simulink library "visionanalysis"  (R2024b)
settings: Solver=ode45  StartTime=0.0  StopTime=10.0  RelTol=1e-3
undefined symbols (not defined in the file or in its folder): dtInfo, fspecial
libraries: visionstatistics x1
(part 2 of 2)

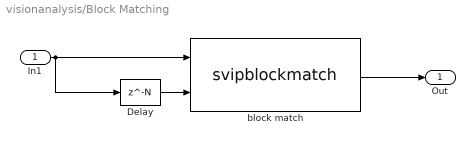
== system visionanalysis/Block Matching ==
  In1 : Inport
  Delay : Delay  DelayLength=N
  block match : S-Function  DialogController=vipDDGCreate  FunctionName=svipblockmatch  Parameters=searchMethod,blockSize,overlapping,maxDisplacement,matchCriteria,outVelForm,dtInfo.prodOutputMode,dtInfo.prodOutputWordLength,dtInfo.prodOutputFracLength,dtInfo.accumMode,dtInfo.accumWordLength,dtInfo.accumFracLength,dtInfo.outputMode,dtInfo.outputWordLength,dtInfo.outputFracLength,dtInfo.roundingMode,dtInfo.overflowMode  SFunctionDeploymentMode=off  EnableBusSupport=off  mask(block match){which2img=Two images, N=1, searchMethod=Exhaustive, blockSize=blockSize, overlapping=overlapping, maxDisplacement=maxDisplacement, matchCriteria=Mean square error (MSE), outVelForm=Magnitude-squared, outputMode=Binary point scaling, outputWordLength=outputWordLength, outputFracLength=outputFracLength, accumMode=Binary point scaling, accumWordLength=accumWordLength, accumFracLength=accumFracLength, prodOutputMode=Binary point scaling, prodOutputWordLength=prodOutputWordLength, prodOutputFracLength=prodOutputFracLength, roundingMode=Floor, overflowMode=on, LockScale=off}
      mask prompts: which2img "Estimate motion between:"; searchMethod "Search method:"; blockSize "Block size [height width]:"; overlapping "Overlap size [r c]:"; maxDisplacement "Maximum displacement [r c]:"; matchCriteria "Block matching criteria:"; outVelForm "Velocity output:"; outputMode "Fixed-point output attributes:"; outputWordLength "Output word length:"; outputFracLength "Output fractional length:"; accumMode "Fixed-point accumulator attributes:"; accumWordLength "Accumulator word length:"; accumFracLength "Accumulator fraction length:"; prodOutputMode "Fixed-point product output attributes:"; prodOutputWordLength "Product output word length:"; prodOutputFracLength "Product output fraction length:"; roundingMode "Round integer calculations towards:"; overflowMode "Saturate on integer overflow"; LockScale "Lock scaling"
      mask help: Estimates motion between two images or two video frames using block matching method.
      mask init:
      | dtInfo = dspGetFixptDataTypeInfo(gcbh,15);
      mask TypeOptions which2img: Two images | Current frame and N-th frame back
      mask TypeOptions searchMethod: Exhaustive | Three-step
      mask TypeOptions matchCriteria: Mean square error (MSE) | Mean absolute difference (MAD)
      mask TypeOptions outVelForm: Horizontal and vertical components in complex form | Magnitude-squared
      mask TypeOptions outputMode: Binary point scaling | Slope and bias scaling
      mask TypeOptions accumMode: Binary point scaling | Slope and bias scaling
      mask TypeOptions prodOutputMode: Same as input | Binary point scaling | Slope and bias scaling
      mask TypeOptions roundingMode: Ceiling | Convergent | Floor | Nearest | Round | Simplest | Zero
  Out : Outport  VectorParamsAs1DForOutWhenUnconnected=off
  wires:
  In1/1 -> block match/1, Delay/1
  block match/1 -> Out/1
  Delay/1 -> block match/2

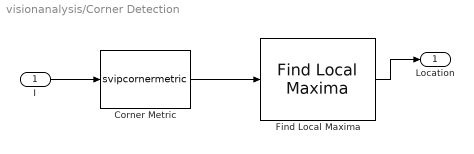
== system visionanalysis/Corner Detection ==
  I : Inport
  Corner Metric : S-Function  FunctionName=svipcornermetric  Parameters=method, factor, filter, thrInten, thrAngle, output, outputInUse, maxNum, thrMetric, neighborSize, dtInfo.firstCoeffMode,dtInfo.firstCoeffWordLength,dtInfo.firstCoeffFracLength,dtInfo. prodOutputMode,dtInfo.prodOutputWordLength,dtInfo.prodOutputFracLength,dtInfo.accumMode,dtInfo.accumWordLength,dtInfo.accumFracLength,dtInfo.memoryMode,dtInfo.memoryWordLength,dtInfo.memoryFracLength,dtInfo.outputMode,dtInfo.outputWordLength,dtInfo.outputFracLength,dtInfo.roundingMode,dtInfo.overflowMode  SFunctionDeploymentMode=off  EnableBusSupport=off  mask(Corner Metric){method=Harris corner detection (Harris & Stephens), factor=factor, filter=reshape([filter(:), filter(:)], [2*length(filter), 1]), thrInten=thrInten, thrAngle=157.5, output=Obsolete9b, outputInUse=Corner location, maxNum=maxNum, thrMetric=thrMetric, neighborSize=neighborSize, isOutVarDim=off, roundingMode=Floor, overflowMode=off, firstCoeffMode=Specify word length, firstCoeffWordLength=firstCoeffWordLength, firstCoeffFracLength=firstCoeffFracLength, firstCoeffSlope=2^-(firstCoeffFracLength), prodOutputMode=Binary point scaling, prodOutputWordLength=prodOutputWordLength, prodOutputFracLength=prodOutputFracLength, prodOutputSlope=2^-(prodOutputFracLength), accumMode=Binary point scaling, accumWordLength=accumWordLength, accumFracLength=accumFracLength, accumSlope=2^-(accumFracLength), memoryMode=Binary point scaling, memoryWordLength=memoryWordLength, memoryFracLength=memoryFracLength, memorySlope=2^-(memoryFracLength), outputMode=Same as accumulator, outputWordLength=outputWordLength, outputFracLength=outputFracLength, outputSlope=2^-(outputFracLength), LockScale=off}
      mask prompts: factor "Sensitivity factor (0<k<0.25):"; filter "Coefficients for separable smoothing filter:"; thrInten "Intensity comparison threshold:"; thrAngle "Maximum angle to be considered a corner (in degrees):"; outputInUse "Output:"; maxNum "Maximum number of corners:"; thrMetric "Minimum metric value that indicates a corner:"; neighborSize "Neighborhood size (suppress region around detected corners):"; isOutVarDim "Output variable size signal"; roundingMode "vision:masks:RoundingMode"; overflowMode "Saturate on integer overflow"; LockScale "Simulink:masks:LockDataTypeAgainstFxpTools_MP"
      mask help: Calculates the corner metric matrix. This is not a stand alone block: please do not change parameters.
      mask init:
      | blkh = gcbh;
      | dtInfo = dspGetFixptDataTypeInfo(blkh, 63);
      mask Help: eval('visionblockhelp');
      mask TypeOptions method: vision:masks:HarrisCornerDetectionHarrisSteph | vision:masks:MinimumEigenvalueShiTomasi | vision:masks:LocalIntensityComparisonRosenDr
      mask Callback method: vipblkcddynamic;
      mask TypeOptions thrAngle: 22.5 | 45.0 | 67.5 | 90.0 | 112.5 | 135.0 | 157.5
      mask TypeOptions output: vision:masks:CornerLocation | vision:masks:CornerLocationAndMetricMatrix | vision:masks:MetricMatrix | vision:masks:Obsolete9b
      mask TypeOptions outputInUse: vision:masks:CornerLocation | vision:masks:CornerLocationAndMetricMatrix | vision:masks:MetricMatrix
      mask Callback outputInUse: vipblkcddynamic;
      mask TypeOptions roundingMode: Simulink:dialog:Ceiling_CB | Simulink:dialog:Convergent_CB | Simulink:dialog:Floor_CB | Simulink:dialog:Nearest_CB | Simulink:dialog:Round_CB | Simulink:dialog:Simplest_CB | Simulink:dialog:Zero_CB
      mask TypeOptions firstCoeffMode: Simulink:dialog:UDTSameAsInputWordLengthRule | vision:masks:SpecifyWordLength | vision:masks:BinaryPointScaling | vision:masks:SlopeAndBiasScaling
      mask Callback firstCoeffMode: vipblkcddynamic;
      mask TypeOptions prodOutputMode: Simulink:dialog:UDTSameAsInputRule | vision:masks:BinaryPointScaling | vision:masks:SlopeAndBiasScaling
      mask Callback prodOutputMode: vipblkcddynamic;
      mask TypeOptions accumMode: Simulink:dialog:UDTSameAsInputRule | vision:masks:BinaryPointScaling | vision:masks:SlopeAndBiasScaling
      mask Callback accumMode: vipblkcddynamic;
      mask TypeOptions memoryMode: Simulink:dialog:UDTSameAsInputRule | vision:masks:BinaryPointScaling | vision:masks:SlopeAndBiasScaling
      mask Callback memoryMode: vipblkcddynamic;
      mask TypeOptions outputMode: Simulink:dialog:UDTSameAsAccumulatorRule | Simulink:dialog:UDTSameAsInputRule | vision:masks:BinaryPointScaling | vision:masks:SlopeAndBiasScaling
      mask Callback outputMode: vipblkcddynamic;
      mask DialogControl Container6 Prompt: vision:masks:Main
      mask DialogControl dataTypesTab Prompt: vision:masks:DataTypes
      mask DialogControl fixptTrumpRule Prompt: Simulink:dialog:FloatingPointTrumpRule
      mask DialogControl fixptOpParams Prompt: vision:masks:FixptOpParams
      mask DialogControl roundingMode Prompt: Rounding mode:
      mask DialogControl fixptDataTypes Prompt: vision:masks:FixptDataTypes
      mask DialogControl openDataTypeDiagram Prompt: vision:masks:OpenDataTypeDiagram
      mask DialogControl dataTypeColumnLabel Prompt: Simulink:dialog:FcnColumnHeaderDataType
      mask DialogControl signedColumnLabel Prompt: Simulink:dialog:UDTSignedSign
      mask DialogControl wordLengthColumnLabel Prompt: Simulink:dialog:UDTWordLengthEdit
      mask DialogControl fractionLengthColumnLabel Prompt: Simulink:dialog:UDTFractionLengthEdit
      mask DialogControl slopeColumnLabel Prompt: Simulink:dialog:UDTSlopeEdit
      mask DialogControl biasColumnLabel Prompt: Simulink:dialog:UDTBiasEdit
      mask DialogControl firstCoeffLabel Prompt: vision:masks:Coefficients
      mask DialogControl firstCoeffSignedText Prompt: Simulink:dialog:Yes_CB
      mask DialogControl firstCoeffBias Prompt: 0
      mask DialogControl prodOutputLabel Prompt: vision:masks:ProductOutput
      mask DialogControl prodOutputSignedText Prompt: Simulink:dialog:Yes_CB
      mask DialogControl prodOutputBias Prompt: 0
      mask DialogControl accumLabel Prompt: vision:masks:Accumulator
      mask DialogControl accumSignedText Prompt: Simulink:dialog:Yes_CB
      mask DialogControl accumBias Prompt: 0
      mask DialogControl memoryLabel Prompt: vision:masks:Memory
      mask DialogControl memorySignedText Prompt: Simulink:dialog:Yes_CB
      mask DialogControl memoryBias Prompt: 0
      mask DialogControl outputLabel Prompt: vision:masks:MetricOutput
      mask DialogControl outputSignedText Prompt: Simulink:dialog:Yes_CB
      mask DialogControl outputBias Prompt: 0
      mask DialogControl LockScale Prompt: Lock data type settings against changes by the fixed-point tools
      mask Display: disp('Corner Metric');
  Find Local Maxima : visionstatistics/Find Local Maxima  num_peaks=maxNum  nhood_size=neighborSize  src_thresh=Obsolete9b  src_thresh_inuse=Specify via dialog  threshold=thrMetric  inputIsHough=off  dt_peak=uint32  isOutVarDim=on  dt_count=uint32
  Location : Outport  VectorParamsAs1DForOutWhenUnconnected=off
  wires:
  I/1 -> Corner Metric/1
  Corner Metric/1 -> Find Local Maxima/1
  Find Local Maxima/1 -> Location/1

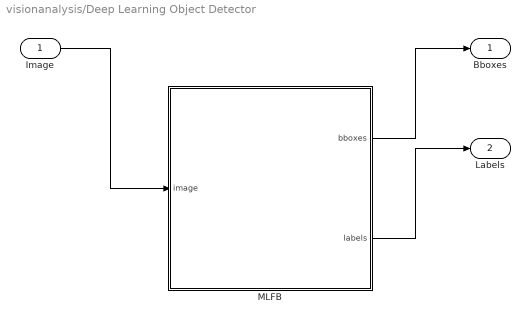
== system visionanalysis/Deep Learning Object Detector ==
  Image : Inport
  MLFB : MATLAB Function  TreatAsAtomicUnit=on
  Bboxes : Outport
  Labels : Outport  Port=2
  wires:
  Image/1 -> MLFB/1(image)
  MLFB/1(bboxes) -> Bboxes/1
  MLFB/2(labels) -> Labels/1

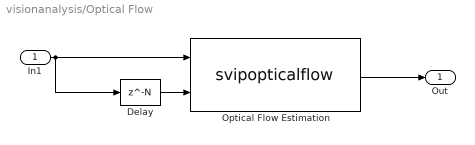
== system visionanalysis/Optical Flow ==
  In1 : Inport
  Delay : Delay  DelayLength=N
  Optical Flow Estimation : S-Function  DialogController=vipDDGCreate  FunctionName=svipopticalflow  Parameters=method,gradMethod,outVelForm,lambda,stop_criteria,maxAllowAbsDiff,maxIter,numInports,sigmaS,sigmaW,eigTh,discardNormalFlow,dtInfo.firstCoeffMode, dtInfo.firstCoeffWordLength,dtInfo.firstCoeffFracLength,dtInfo.prodOutputMode,dtInfo.prodOutputWordLength,dtInfo.prodOutputFracLength,dtInfo.accumMode,dtInfo.accumWordLength,dtInfo.accumFracLength,dtInfo.memoryMode,dtInfo.memoryWordLength,dtInfo.memoryFracLength,dtInfo.outputMode,dtInfo.outputWordLength,dtInfo.outputFracLength,dtInfo.roundingMode,dtInfo.overflowMode  SFunctionDeploymentMode=off  EnableBusSupport=off  mask(Optical Flow Estimation){method=Horn-Schunck, gradMethod=Difference filter [-1 1], which2img=Current frame and N-th frame back, N=N, outVelForm=Magnitude-squared, lambda=lambda, stop_criteria=When maximum number of iterations is reached, maxAllowAbsDiff=maxAllowAbsDiff, maxIter=maxIter, numInports=numInports, sigmaS=sigmaS, sigmaW=sigmaW, eigTh=eigTh, discardNormalFlow=off, outputCurrentImage=off, firstCoeffMode=Same word length as first input, firstCoeffWordLength=firstCoeffWordLength, firstCoeffFracLength=firstCoeffFracLength, prodOutputMode=Binary point scaling, prodOutputWordLength=prodOutputWordLength, prodOutputFracLength=prodOutputFracLength, accumMode=Same as product output, accumWordLength=accumWordLength, accumFracLength=accumFracLength, memoryMode=Same as accumulator, memoryWordLength=memoryWordLength, memoryFracLength=memoryFracLength, outputMode=Binary point scaling, outputWordLength=outputWordLength, outputFracLength=outputFracLength, roundingMode=Nearest, overflowMode=on, LockScale=off}
      mask prompts: gradMethod "Gradient method:"; which2img "Compute optical flow between:"; outVelForm "Velocity output:"; lambda "Smoothness factor:"; stop_criteria "Stop iterative solution:"; maxAllowAbsDiff "Velocity difference threshold:"; maxIter "Maximum number of iterations:"; numInports "Number of input frames to buffer:"; sigmaS "Standard deviation for image smoothing filter:"; sigmaW "Standard deviation for gradient smoothing filter:"; eigTh "Threshold for noise reduction:"; discardNormalFlow "Discard normal flow estimates when constraint equation is ill-conditioned"; outputCurrentImage "Output image corresponding to motion vectors (accounts for block delay)"; firstCoeffMode "Eigen threshold attributes:"; firstCoeffWordLength "Eigen threshold word length:"; firstCoeffFracLength "Eigen threshold fraction length:"; prodOutputMode "Product output attributes:"; prodOutputWordLength "Product output word length:"; prodOutputFracLength "Product output fraction length:"; accumMode "Accumulator attributes:"; accumWordLength "Accumulator word length:"; accumFracLength "Accumulator fraction length:"; memoryMode "Gradient attributes:"; memoryWordLength "Gradient word length:"; memoryFracLength "Gradient fraction length:"; outputMode "Fixed-point output attributes:"; outputWordLength "Output word length:"; outputFracLength "Output fractional length:"; roundingMode "Round integer calculations toward:"; overflowMode "Saturate on integer overflow"; LockScale "Lock scaling"
      mask help: Estimates optical flow between two images or two video frames.
      mask init:
      | dtInfo = dspGetFixptDataTypeInfo(gcbh,63);
      mask TypeOptions method: vision:masks:HornSchunck | vision:masks:LucasKanade
      mask TypeOptions gradMethod: vision:masks:DerivativeOfGaussian | vision:masks:DifferenceFilter
      mask TypeOptions which2img: vision:masks:TwoImages | vision:masks:CurrentFrameAndNthFrameBack
      mask TypeOptions outVelForm: vision:masks:HorizontalAndVerticalComponentsI | vision:masks:Magnitudesquared
      mask TypeOptions stop_criteria: vision:masks:WhenVelocityDifferenceFallsBelow | vision:masks:WhenMaximumNumberOfIterations | vision:masks:WhicheverComesFirst
      mask TypeOptions firstCoeffMode: Same word length as first input | Specify word length | Binary point scaling | Slope and bias scaling
      mask TypeOptions prodOutputMode: Binary point scaling | Slope and bias scaling
      mask TypeOptions accumMode: Same as product output | Binary point scaling | Slope and bias scaling
      mask TypeOptions memoryMode: Same as accumulator | Same as product output | Binary point scaling | Slope and bias scaling
      mask TypeOptions outputMode: Binary point scaling | Slope and bias scaling
      mask TypeOptions roundingMode: Ceiling | Convergent | Floor | Nearest | Round | Simplest | Zero
  Out : Outport  VectorParamsAs1DForOutWhenUnconnected=off
  wires:
  Optical Flow Estimation/1 -> Out/1
  In1/1 -> Optical Flow Estimation/1, Delay/1
  Delay/1 -> Optical Flow Estimation/2

== matlab function visionanalysis/Deep Learning Object Detector/MLFB ==
  data: image input; bboxes output; labels output
function [bboxes, labels] = detect(image)
[bboxes, labels] = deep.blocks.internal.detector(image, 'untitled.mat', [], 0.5, 2000, [], [], 10, true, false, true);
end
